simulink model "rvs_testing"  (R2014b)
settings: Solver=ode45  StartTime=0.0  StopTime=10.0  RelTol=1e-3
libraries: rvs x2
settings Model: Creator=Arthur  LastModifiedBy=Arthur

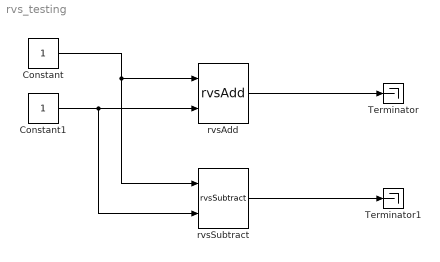
== system rvs_testing ==
  Constant : Constant
  Constant1 : Constant
  Terminator : Terminator
  Terminator1 : Terminator
  rvsAdd : rvs/rvsAdd
  rvsSubtract : rvs/rvsSubtract
  wires:
  Constant1/1 -> rvsSubtract/2, rvsAdd/2
  rvsAdd/1 -> Terminator/1
  Constant/1 -> rvsSubtract/1, rvsAdd/1
  rvsSubtract/1 -> Terminator1/1
